simulink model "Beam_elastic_Coulomb_multisine"  (R2018a)
settings: Solver=FixedStepAuto  StartTime=0.0  StopTime=simtime  FixedStep=step_size  RelTol=1e-7  EnableMultiTasking=on
values from neighbouring files (symbols this model uses):
  A = [zeros(n,n), eye(n) ... (first row only)    [Beam_ealstic_Coulomb_NMA.m]
  A_shaker = [- R/L 0 -Tau/L 0 0; 0 0 1 0 0;      Tau/M_C -K_C/M_C -C_C/M_C K_C/M_C C_C/M_C; 0 0 0 0 1;      0 K_C/M_T C_C/M_T -(K_C+K_S)/M_T -(C_C+C_S)/M_T]    [Beam_ealstic_Coulomb_NMA.m]
  B = [zeros(n,1);beam.M\loc_exc]    [Beam_ealstic_Coulomb_NMA.m]    (also in beam_frf.m = eye(length(beam.M)); B(:,inl) = [])
  B_nl = [zeros(n,1);beam.M\loc_nl]    [Beam_ealstic_Coulomb_NMA.m]
  B_shaker = [Tau/M_C 0 0 0 0; 0 0 0 0 1/M_T]'    [Beam_ealstic_Coulomb_NMA.m]
  C_shaker = [0 0 0 1 0; 0 0 0 0 1]    [Beam_ealstic_Coulomb_NMA.m]
  k_stinger = (E_stinger*A_stinger)/l_stinger    (= 131946891.451)    [Beam_ealstic_Coulomb_NMA.m]
  kt = 1.3e6    (= 1300000)    [Beam_ealstic_Coulomb_NMA.m]    (also in beam_frf.m; beam_nma.m; nidish_1.m)
  muN = 1    [Beam_ealstic_Coulomb_NMA.m]    (also in beam_frf.m; beam_nma.m; nidish_1.m)
  T_disp = [eye(n,n) zeros(n,n)]    [Beam_ealstic_Coulomb_NMA.m]
  T_exc = zeros(1,2*n)    [Beam_ealstic_Coulomb_NMA.m]
  T_nl = zeros(1,2*n)    [Beam_ealstic_Coulomb_NMA.m]    (also in beam_frf.m = beam.nonlinear_elements{1}.force_direction'; beam_plot.m = beam.nonlinear_elements{1}.force_direction')
  x0beam = 0    [Beam_ealstic_Coulomb_NMA.m]
libraries: simulink x1
settings Model: SimulationMode=accelerator  Creator=peter  LastModifiedBy=paw
settings SolverCC: ZeroCrossAlgorithm=Adaptive  SolverResetMethod=Robust
settings DataIOCC: LimitDataPoints=on  SaveFormat=Array  SignalLoggingSaveFormat=ModelDataLogs
settings OptimizationCC: LifeSpan=inf
settings DebuggingCC: UnderspecifiedInitializationDetection=Classic  MergeDetectMultiDrivingBlocksExec=none  SolverPrmCheckMsg=warning  MultiTaskDSMMsg=warning  MultiTaskCondExecSysMsg=none  StateNameClashWarn=warning  SFUnexpectedBacktrackingDiag=warning  SFNoUnconditionalDefaultTransitionDiag=warning  SFExecutionAtInitializationDiag=none
settings HardwareCC: ProdBitPerPointer=32  ProdBitPerSizeT=32  ProdBitPerPtrDiffT=32  ProdLargestAtomicFloat=None  ProdIntDivRoundTo=Undefined  ProdEndianess=Unspecified  ProdWordSize=32  ProdHWDeviceType=32-bit Generic
settings ModelReferenceCC: UpdateModelReferenceTargets=IfOutOfDate  PropagateSignalLabelsOutOfModel=off
settings SFSimCC: SFSimEcho=off
settings CodeAppCC: StateflowObjectComments=on
settings GRTTargetCC: TargetLangStandard=C89/C90 (ANSI)  GeneratePreprocessorConditionals=Disable all
settings ConfigComp: CovMetricSettings=dw  CovHtmlReporting=on  CovSaveCumulativeToWorkspaceVar=on  CovSaveSingleToWorkspaceVar=on  CovExternalEMLEnable=off
settings SimscapeCC: SimscapeNormalizeSystem=off

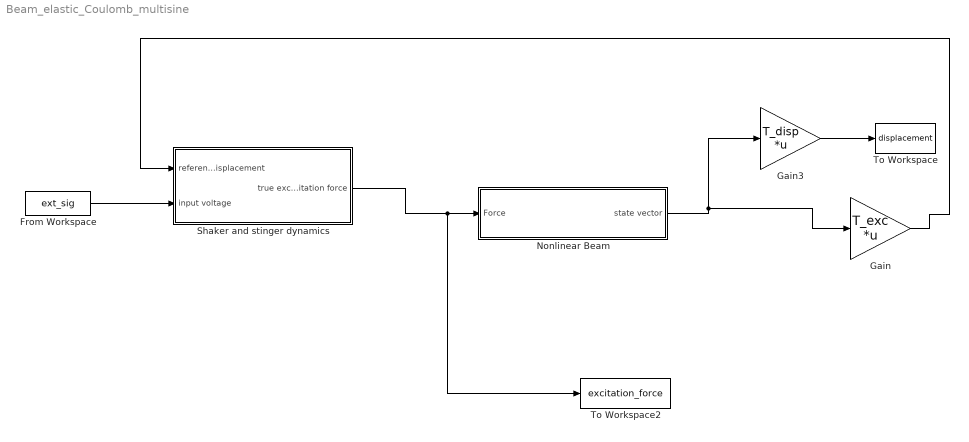
== system Beam_elastic_Coulomb_multisine ==
  From Workspace : FromWorkspace  VariableName=ext_sig  SampleTime=0
  Gain : Gain  Gain=T_exc  Multiplication=Matrix(K*u)
  Gain3 : Gain  Gain=T_disp  Multiplication=Matrix(K*u)
  Nonlinear Beam : Subsystem
  Shaker and stinger dynamics : Subsystem
  To Workspace : ToWorkspace  VariableName=displacement  SaveFormat=Structure With Time  SampleTime=-1
  To Workspace2 : ToWorkspace  VariableName=excitation_force  SaveFormat=Structure With Time  SampleTime=-1
  wires:
  Nonlinear Beam/1(state vector) -> Gain/1, Gain3/1
  Gain/1 -> Shaker and stinger dynamics/1(reference displacement)
  Shaker and stinger dynamics/1(true excitation force) -> To Workspace2/1, Nonlinear Beam/1(Force)
  Gain3/1 -> To Workspace/1
  From Workspace/1 -> Shaker and stinger dynamics/2(input voltage)

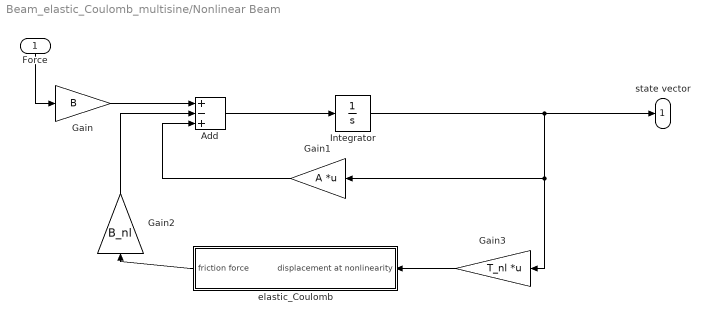
== system Beam_elastic_Coulomb_multisine/Nonlinear Beam ==
  Force : Inport
  Add : Sum  Inputs=+-+
  Gain : Gain  Gain=B
  Gain1 : Gain  Gain=A  Multiplication=Matrix(K*u) (u vector)
  Gain2 : Gain  Gain=B_nl
  Gain3 : Gain  Gain=T_nl  Multiplication=Matrix(K*u)
  Integrator : Integrator  InitialCondition=x0beam
  elastic_Coulomb : Subsystem
  state vector : Outport
  wires:
  Force/1 -> Gain/1
  Gain/1 -> Add/1
  Add/1 -> Integrator/1
  Integrator/1 -> Gain3/1, Gain1/1, state vector/1
  Gain1/1 -> Add/3
  Gain2/1 -> Add/2
  elastic_Coulomb/1(friction force) -> Gain2/1
  Gain3/1 -> elastic_Coulomb/1(displacement at nonlinearity)

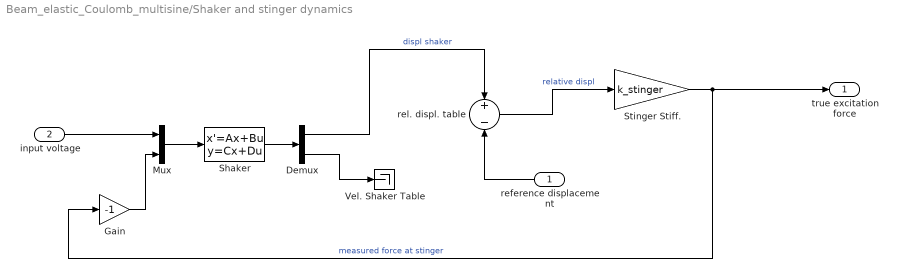
== system Beam_elastic_Coulomb_multisine/Shaker and stinger dynamics ==
  reference displacement : Inport
  input voltage : Inport  Port=2
  Demux : Demux  Outputs=2
  Gain : Gain  Gain=-1
  Mux : Mux  Inputs=2
  Shaker : StateSpace  A=A_shaker  B=B_shaker  C=C_shaker  D=[0 0;0 0]  InitialCondition=0
  Stinger Stiff. : Gain  Gain=k_stinger
  Vel. Shaker Table : Terminator
  rel. displ. table : Sum  Inputs=+-
  true excitation force : Outport
  wires:
  Stinger Stiff./1 -> Gain/1, true excitation force/1  "measured force at stinger"
  rel. displ. table/1 -> Stinger Stiff./1  "relative displ"
  Shaker/1 -> Demux/1
  Demux/1 -> rel. displ. table/1  "displ shaker"
  Demux/2 -> Vel. Shaker Table/1
  reference displacement/1 -> rel. displ. table/2
  Gain/1 -> Mux/2
  input voltage/1 -> Mux/1
  Mux/1 -> Shaker/1

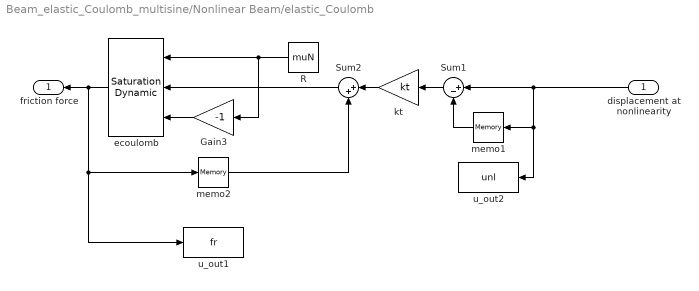
== system Beam_elastic_Coulomb_multisine/Nonlinear Beam/elastic_Coulomb ==
  displacement at nonlinearity : Inport
  Gain3 : Gain  Gain=-1
  R : Constant  Value=muN
  Sum1 : Sum  Inputs=|+-
  Sum2 : Sum  Inputs=|++
  ecoulomb : simulink/Discontinuities/Saturation Dynamic  OutMin=[]  OutMax=[]  OutDataTypeStr=Inherit: Same as second input  OutDataType=fixdt(1, 16)  OutScaling=2^-10  DoSatur=off
  kt : Gain  Gain=kt
  memo1 : Memory
  memo2 : Memory
  u_out1 : ToWorkspace  VariableName=fr  SampleTime=-1
  u_out2 : ToWorkspace  VariableName=unl  SampleTime=-1
      settings: MaxDataPoints=1
  friction force : Outport
  wires:
  Sum1/1 -> kt/1
  kt/1 -> Sum2/1
  R/1 -> ecoulomb/1, Gain3/1
  Gain3/1 -> ecoulomb/3
  Sum2/1 -> ecoulomb/2
  ecoulomb/1 -> friction force/1, u_out1/1, memo2/1
  memo2/1 -> Sum2/2
  displacement at nonlinearity/1 -> Sum1/1, memo1/1, u_out2/1
  memo1/1 -> Sum1/2
